simulink model "PWM"  (R2018a)
settings: Solver=VariableStepAuto  StartTime=0.0  StopTime=8  RelTol=1e-3
libraries: elec_lib x6, fl_lib x4, nesl_utility x4
settings Model: Creator=Oscar  LastModifiedBy=Oscar

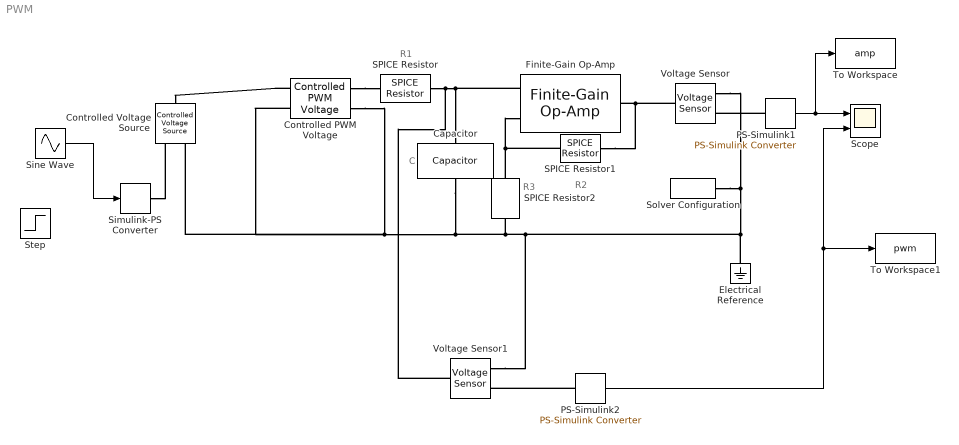
== system PWM ==
  note: C
  note: R2
  note: R3
  note: R1
  Capacitor : elec_lib/Passive Devices/Capacitor  enable_table=0  c=10 uF  Cvec=[1e-05, 1e-06] F  Vvec=[0, 10] V  CV_table_symmetry=1  C_tol=5  enable_C_tol=0  tol_distribution=1  nSigma=4  r=1e-6 Ohm  g=0 1/Ohm  enable_operating_limits=0  operating_limit_action=2  max_working_voltage_range=[-25, 25] V  power_rating=1 W  enable_faults=0  fault_action=1  Cscale_faulted=100  R_faulted=1e-3 Ohm  G_faulted=0 1/Ohm  tau_fault=1e-3 s  enable_temporal_fault=0  t_fault=1 s  enable_behavioral_fault=0  max_permissible_voltage_range=[-100, 100] V  t_fail_on_voltage=1 s  i_specify=off  i_priority=None  i=0 A  i_nominal_specify=off  i_nominal_unit=A  i_nominal_value=1  v_specify=off  v_priority=None  v=0 V  v_nominal_specify=off  v_nominal_unit=V  v_nominal_value=1  vc_specify=off  vc_priority=High  vc=0 V  vc_nominal_specify=off  vc_nominal_unit=V  vc_nominal_value=1
  Controlled PWM Voltage : elec_lib/Actuators & Drivers/Drivers/Controlled PWM Voltage  F=1 kHz  TD=0 s  pulse_width_offset=0 s  pulse_min=0 s  Vmin=0 V  Vmax=5 V  Vm=3.3 V  pwm_or_av=1  event_type=1  sample_time=1e-6 s  u_min=0  u_max=1
      settings: SourceProductName=Simscape Electronics  SourceProductBaseCode=SN
  Controlled Voltage Source : fl_lib/Electrical/Electrical Sources/Controlled Voltage Source
  Electrical Reference : fl_lib/Electrical/Electrical Elements/Electrical Reference
  Finite-Gain Op-Amp : elec_lib/Integrated Circuits/Finite-Gain Op-Amp  A=1000  Rin=1e6 Ohm  Rout=100 Ohm  Vmin=-100 V  Vmax=100 V  noise_mode=0  v_noise=30e-9 V/Hz^0.50000  noise_prm=1  i_noise=0.5e-12 A/Hz^0.50000  ip_noise=0.5e-12 A/Hz^0.50000  in_noise=0.5e-12 A/Hz^0.50000  sample_time=1e-3 s  repeatability=1  auto_seed_v=2868319722  auto_seed_ip=3626636697  auto_seed_in=1479454791  user_seed_v=0  user_seed_ip=0  user_seed_in=0
      settings: SourceProductName=Simscape Electronics  SourceProductBaseCode=SN
  PS-Simulink1 : nesl_utility/PS-Simulink Converter  PhysicalDomain=network_engine_domain  SubClassName=ps_output  LeftPortType=input  RightPortType=output  PseudoPeriodic=off  Frequencies=[]  Unit=V  AffineConversion=off
  PS-Simulink2 : nesl_utility/PS-Simulink Converter  PhysicalDomain=network_engine_domain  SubClassName=ps_output  LeftPortType=input  RightPortType=output  PseudoPeriodic=off  Frequencies=[]  Unit=V  AffineConversion=off
  SPICE Resistor : elec_lib/Additional Components/SPICE-Compatible Components/Passive Devices/SPICE Resistor  SCALE=1.0  R_param=1  R=1.3 kOhm  RSH=0 Ohm  LENGTH=1e-6 m  WIDTH=1e-6 m  NARROW=0 m  T_param=1  TC1=0 1/K  TC2=0 1/K^2  TOFFSET=0 K  TFIXED=300.15 K  TMEAS=300.15 K
      settings: SourceProductName=Simscape Electronics  SourceProductBaseCode=SN
  SPICE Resistor1 : elec_lib/Additional Components/SPICE-Compatible Components/Passive Devices/SPICE Resistor  SCALE=1.0  R_param=1  R=240 Ohm  RSH=0 Ohm  LENGTH=1e-6 m  WIDTH=1e-6 m  NARROW=0 m  T_param=1  TC1=0 1/K  TC2=0 1/K^2  TOFFSET=0 K  TFIXED=300.15 K  TMEAS=300.15 K
      settings: SourceProductName=Simscape Electronics  SourceProductBaseCode=SN
  SPICE Resistor2 : elec_lib/Additional Components/SPICE-Compatible Components/Passive Devices/SPICE Resistor  SCALE=1.0  R_param=1  R=118 Ohm  RSH=0 Ohm  LENGTH=1e-6 m  WIDTH=1e-6 m  NARROW=0 m  T_param=1  TC1=0 1/K  TC2=0 1/K^2  TOFFSET=0 K  TFIXED=300.15 K  TMEAS=300.15 K
      settings: SourceProductName=Simscape Electronics  SourceProductBaseCode=SN
  Scope : Scope  NumInputPorts=2
  Simulink-PS Converter : nesl_utility/Simulink-PS Converter  PhysicalDomain=network_engine_domain  SubClassName=ps_input  LeftPortType=input  RightPortType=output  PseudoPeriodic=off  Frequencies=[]  NoiseDistribution=none  NoiseParameters=[]  Unit=1  AffineConversion=off  FilteringAndDerivatives=provide  SimscapeFilterOrder=1  InputFilterTimeConstant=0.001  UdotUserProvided=0
  Sine Wave : Sin  Amplitude=2.5  Bias=2.5  Frequency=pi/2  Phase=-pi/2  SampleTime=0
  Solver Configuration : nesl_utility/Solver Configuration  PhysicalDomain=network_engine_domain  SubClassName=solver  LeftPortType=input  RightPortType=generic  Tones=[]  Harmonics=[]  SimulateNoise=off  Profile=off  UseLocalSampling=off  EnableSwitchedLinearOptims=on  FrequencyDomain=off  UseCCode=off  RelTol=0.001  AbsTol=1e-06  MinStep=1e-09  ToWorkspace=off  RevertToSquareIcSolve=off  NumHomotopyIterations=100  PhasorMode=off  PhasorModeNumHarmonics=1  DoDC=off  ResidualTolerance=1e-9  UseLocalSolver=off  LocalSolverChoice=NE_BACKWARD_EULER_ADVANCER  LocalSolverSampleTime=.001  DoFixedCost=off  MaxNonlinIter=3  MaxModeIter=2  LinearAlgebra=Sparse  EquationFormulation=NE_TIME_EF  DelaysMemoryBudget=1024  AutomaticFiltering=on  FilteringTimeConstant=0.001
  Step : Step  Time=0  After=5  SampleTime=0
  To Workspace : ToWorkspace  VariableName=amp  SaveFormat=Timeseries  SampleTime=-1
  To Workspace1 : ToWorkspace  VariableName=pwm  SaveFormat=Timeseries  SampleTime=-1
  Voltage Sensor : fl_lib/Electrical/Electrical Sensors/Voltage Sensor
  Voltage Sensor1 : fl_lib/Electrical/Electrical Sensors/Voltage Sensor
  wires:
  PS-Simulink1/1 -> To Workspace/1, Scope/1
  PS-Simulink2/1 -> To Workspace1/1, Scope/2
  Sine Wave/1 -> Simulink-PS Converter/1
  connections:
  SPICE Resistor/RConn1 -- Voltage Sensor1/LConn1 -- Finite-Gain Op-Amp/LConn1 -- Capacitor/LConn1
  Voltage Sensor/RConn2 -- Solver Configuration/RConn1 -- Electrical Reference/LConn1 -- Voltage Sensor1/RConn2 -- Controlled Voltage Source/RConn2 -- Controlled PWM Voltage/LConn2 -- Controlled PWM Voltage/RConn2 -- Capacitor/RConn1 -- SPICE Resistor2/RConn1
  SPICE Resistor1/LConn1 -- Voltage Sensor/LConn1 -- Finite-Gain Op-Amp/RConn1
  SPICE Resistor2/LConn1 -- SPICE Resistor1/RConn1 -- Finite-Gain Op-Amp/LConn2
  PS-Simulink1/LConn1 -- Voltage Sensor/RConn1
  Controlled PWM Voltage/RConn1 -- SPICE Resistor/LConn1
  Controlled PWM Voltage/LConn1 -- Controlled Voltage Source/LConn1
  Simulink-PS Converter/RConn1 -- Controlled Voltage Source/RConn1
  PS-Simulink2/LConn1 -- Voltage Sensor1/RConn1
